simulink model "dyn_zlin_mod_dyskretny"  (R2014b)
settings: Solver=ode45  StartTime=0.0  StopTime=tkonc  RelTol=1e-3
undefined symbols (not defined in the file): a1, a2, a3, a4, K, T1, T2, Tp, U, x0
settings Model: Creator=Konrad  LastModifiedBy=Konrad

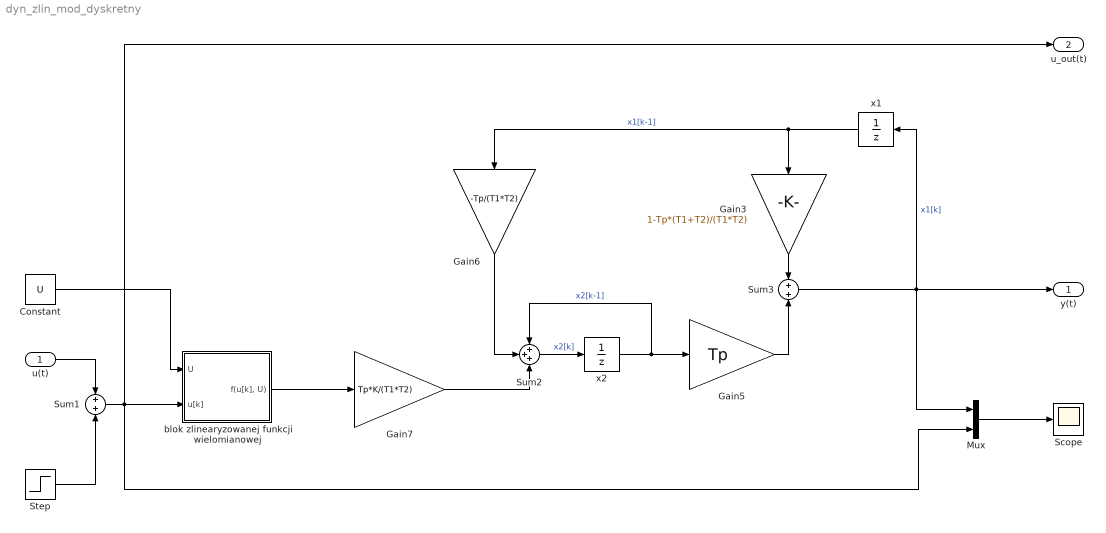
== system dyn_zlin_mod_dyskretny ==
  u(t) : Inport
  Constant : Constant  Value=U
  Gain3 : Gain  Gain=1-Tp*(T1+T2)/(T1*T2)
  Gain5 : Gain  Gain=Tp
  Gain6 : Gain  Gain=-Tp/(T1*T2)
  Gain7 : Gain  Gain=Tp*K/(T1*T2)
  Mux : Mux  Inputs=2
  Scope : Scope
  Step : Step  Time=step(1)  Before=step(2)  After=step(3)  SampleTime=0
  Sum1 : Sum  Inputs=+|+
  Sum2 : Sum  Inputs=+++
  Sum3 : Sum  Inputs=+|+
  blok zlinearyzowanej funkcji wielomianowej : Subsystem
  x1 : UnitDelay  InitialCondition=x0(1)  SampleTime=Tp
  x2 : UnitDelay  InitialCondition=x0(2)  SampleTime=Tp
  y(t) : Outport
  u_out(t) : Outport  Port=2
  wires:
  Sum3/1 -> y(t)/1, Mux/1, x1/1  "x1[k]"
  x1/1 -> Gain6/1, Gain3/1  "x1[k-1]"
  Gain3/1 -> Sum3/1
  x2/1 -> Sum2/1, Gain5/1  "x2[k-1]"
  Gain5/1 -> Sum3/2
  Sum2/1 -> x2/1  "x2[k]"
  Gain6/1 -> Sum2/2
  Gain7/1 -> Sum2/3
  Constant/1 -> blok zlinearyzowanej funkcji wielomianowej/1(U)
  Mux/1 -> Scope/1
  blok zlinearyzowanej funkcji wielomianowej/1("f(u[k], U)") -> Gain7/1
  Sum1/1 -> u_out(t)/1, Mux/2, blok zlinearyzowanej funkcji wielomianowej/2(u[k])
  Step/1 -> Sum1/2
  u(t)/1 -> Sum1/1

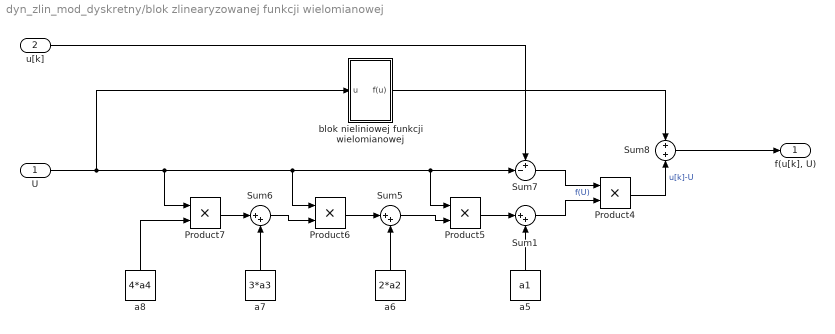
== system dyn_zlin_mod_dyskretny/blok zlinearyzowanej funkcji wielomianowej ==
  U : Inport
  u[k] : Inport  Port=2
  Product{4..7} (4 alike) : Product
  Sum1 : Sum  Inputs=|++
  Sum5 : Sum  Inputs=|++
  Sum6 : Sum  Inputs=|++
  Sum7 : Sum  Inputs=+-|
  Sum8 : Sum
  a5 : Constant  Value=a1
  a6 : Constant  Value=2*a2
  a7 : Constant  Value=3*a3
  a8 : Constant  Value=4*a4
  blok nieliniowej funkcji wielomianowej : Subsystem
  "f(u[k], U)" : Outport
  wires:
  U/1 -> blok nieliniowej funkcji wielomianowej/1(u), Product5/1, Sum7/2, Product6/1, Product7/1
  Product5/1 -> Sum1/1
  Product6/1 -> Sum5/1
  Product7/1 -> Sum6/1
  a5/1 -> Sum1/2
  a6/1 -> Sum5/2
  Sum5/1 -> Product5/2
  a7/1 -> Sum6/2
  Sum6/1 -> Product6/2
  a8/1 -> Product7/2
  Sum1/1 -> Product4/2  "f(U)"
  Sum7/1 -> Product4/1
  u[k]/1 -> Sum7/1
  Product4/1 -> Sum8/2  "u[k]-U"
  Sum8/1 -> "f(u[k], U)"/1
  blok nieliniowej funkcji wielomianowej/1(f(u)) -> Sum8/1

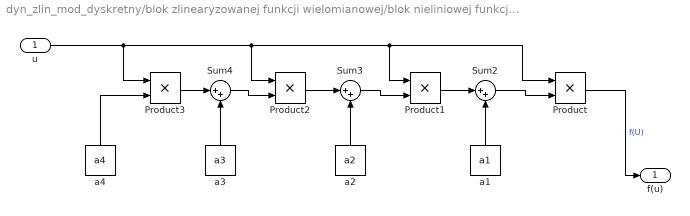
== system dyn_zlin_mod_dyskretny/blok zlinearyzowanej funkcji wielomianowej/blok nieliniowej funkcji wielomianowej ==
  u : Inport
  Product{,1..3} (4 alike) : Product
  Sum2 : Sum  Inputs=|++
  Sum3 : Sum  Inputs=|++
  Sum4 : Sum  Inputs=|++
  a1 : Constant  Value=a1
  a2 : Constant  Value=a2
  a3 : Constant  Value=a3
  a4 : Constant  Value=a4
  f(u) : Outport
  wires:
  u/1 -> Product/1, Product1/1, Product2/1, Product3/1
  Product2/1 -> Sum3/1
  Sum2/1 -> Product/2
  Product/1 -> f(u)/1  "f(U)"
  Product3/1 -> Sum4/1
  a1/1 -> Sum2/2
  a2/1 -> Sum3/2
  Sum3/1 -> Product1/2
  Sum4/1 -> Product2/2
  a3/1 -> Sum4/2
  a4/1 -> Product3/2
  Product1/1 -> Sum2/1
